simulink model "adc16x250"  (R2013b)
settings: Solver=ode45  StartTime=0.0  StopTime=10.0  RelTol=1e-3
libraries: xbsIndex_r4 x23, xps_library x1
settings Model: Creator=root  LastModifiedBy=root

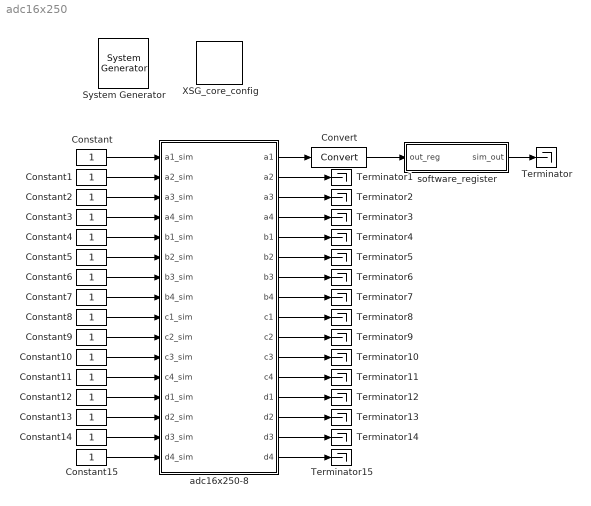
== system adc16x250 ==
  " System Generator" : xbsIndex_r4/ System Generator  Tag=genX  xilinxfamily=virtex6  part=xc6vsx475t  speed=-1  package=ff1759  synthesis_tool=XST  clock_wrapper=Clock Enables  directory=./adc16x250/sysgen  proj_type=Project Navigator  Synth_file=XST Defaults  Impl_file=ISE Defaults  testbench=off  simulink_period=1  sysclk_period=5  dcm_input_clock_period=100  incr_netlist=off  trim_vbits=Everywhere in SubSystem  dbl_ovrd=According to Block Masks  core_generation=According to Block Masks  run_coregen=off  deprecated_control=off  eval_field=0  block_type=sysgen
  Constant{,1..15} (16 alike) : Constant
  Convert : xbsIndex_r4/Convert  gui_display_data_type=Fixed-point  arith_type=Unsigned  n_bits=32  bin_pt=0  float_type=Single  exp_bits=8  fraction_bits=24  quantization=Truncate  overflow=Wrap  en=off  latency=2  dbl_ovrd=off  pipeline=off  block_type=convert
      settings: block_version=11.4
  Terminator{,1..15} (16 alike) : Terminator
  XSG_core_config : xps_library/XSG_core_config  Tag=xps:xsg  hw_sys=ROACH2:sx475t  clk_src=adc0_clk  ROACH_clk_src=sys_clk  ROACH2_clk_src=adc0_clk  MKDIG_clk_src=sys_clk  clk_rate=135  sample_period=1  synthesis_tool=XST
  adc16x250-8 : Subsystem  Tag=xps:adc16  AncestorBlock=xps_library/ADCs/adc16x250-8  mask(ADC16){board_count=1, roach2_rev=2, zdok_rev=2}
      mask prompts: board_count "Number of ADC16 Boards"; roach2_rev "ROACH2 Revision"; zdok_rev "ZDOK Pinout Revision"
      mask help: 16-input ADC. When using one ADC16 board, it must be in ZDOK0.
      mask init:
      | % Only board_count is needed by init function
      | adc16_init(gcb, ...
      |     'board_count', board_count);
      settings: AttributesFormatString=r2 rev%<roach2_rev>\nzdok rev%<zdok_rev>
      mask Help:
      | This is the CASPER "yellow block" for the CASPER ADC16 board.  Each ADC
      | board has four ADC chips.  Each ADC chip accepts four inputs.  The four
      | 8-bit outputs from each ADC chip are concatenated into a 32-bit signal.
      mask TypeOptions board_count: 1 | 2
      mask TypeOptions roach2_rev: 1 | 2
      mask TypeOptions zdok_rev: 1 | 2
  software_register : Subsystem  Tag=xps:sw_reg  AncestorBlock=xps_library/software_register  mask(swreg){io_dir=To Processor, io_delay=0, sample_period=1, names=reg, bitwidths=32, bin_pts=0, arith_types=0, sim_port=on, show_format=on}
      mask prompts: io_dir "I/O direction"; io_delay "I/O delay"; sample_period "Sample period"; names "Bitfield names [msb...lsb]"; bitwidths "Bitfield widths"; bin_pts "Bitfield binary pts"; arith_types "Bitfield types, ufix=0, fix=1, bool=2"; sim_port "Provide sim input/output?"; show_format "Print format string?"
      mask help: A 32-bit software-accessible register. Can be divided into bitfields of varying widths and types using the fields in the block mask.
      mask init:
      | try
      |     swreg_init(gcb)
      | catch ex
      |     disp(sprintf('%s: %s', gcb, ex.message))
      |     errordlg(ex.message)
      | end
      settings: AttributesFormatString=1output:uf32.0 = 32 bits
      mask TypeOptions io_dir: To Processor | From Processor
      mask Callback io_dir:
      | mask_enables = get_param(gcb, 'MaskEnables');
      | mask_names = get_param(gcb, 'MaskNames');
      | if strcmp(get_param(gcb, 'io_dir'), 'To Processor'),
      |     mask_enables{ismember(mask_names, 'sample_period')} = 'off';
      | else
      |     mask_enables{ismember(mask_names, 'sample_period')} = 'on';
      | end
      | set_param(gcb, 'MaskEnables', mask_enables);
  wires:
  adc16x250-8/1(a1) -> Convert/1
  Convert/1 -> software_register/1(out_reg)
  software_register/1(sim_out) -> Terminator/1
  adc16x250-8/2(a2) -> Terminator1/1
  adc16x250-8/3(a3) -> Terminator2/1
  adc16x250-8/4(a4) -> Terminator3/1
  adc16x250-8/5(b1) -> Terminator4/1
  adc16x250-8/6(b2) -> Terminator5/1
  adc16x250-8/7(b3) -> Terminator6/1
  adc16x250-8/8(b4) -> Terminator7/1
  adc16x250-8/9(c1) -> Terminator8/1
  adc16x250-8/10(c2) -> Terminator9/1
  adc16x250-8/11(c3) -> Terminator10/1
  adc16x250-8/12(c4) -> Terminator11/1
  adc16x250-8/13(d1) -> Terminator12/1
  adc16x250-8/14(d2) -> Terminator13/1
  adc16x250-8/15(d3) -> Terminator14/1
  adc16x250-8/16(d4) -> Terminator15/1
  Constant/1 -> adc16x250-8/1(a1_sim)
  Constant1/1 -> adc16x250-8/2(a2_sim)
  Constant3/1 -> adc16x250-8/4(a4_sim)
  Constant2/1 -> adc16x250-8/3(a3_sim)
  Constant5/1 -> adc16x250-8/6(b2_sim)
  Constant7/1 -> adc16x250-8/8(b4_sim)
  Constant6/1 -> adc16x250-8/7(b3_sim)
  Constant4/1 -> adc16x250-8/5(b1_sim)
  Constant8/1 -> adc16x250-8/9(c1_sim)
  Constant9/1 -> adc16x250-8/10(c2_sim)
  Constant11/1 -> adc16x250-8/12(c4_sim)
  Constant10/1 -> adc16x250-8/11(c3_sim)
  Constant13/1 -> adc16x250-8/14(d2_sim)
  Constant15/1 -> adc16x250-8/16(d4_sim)
  Constant14/1 -> adc16x250-8/15(d3_sim)
  Constant12/1 -> adc16x250-8/13(d1_sim)

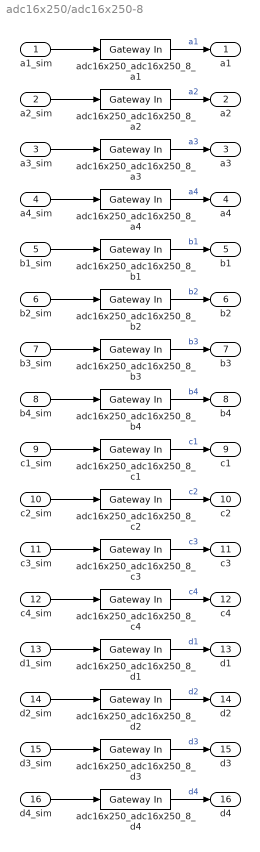
== system adc16x250/adc16x250-8 ==
  a1_sim : Inport
  a2_sim : Inport  Port=2
  a3_sim : Inport  Port=3
  a4_sim : Inport  Port=4
  b1_sim : Inport  Port=5
  b2_sim : Inport  Port=6
  b3_sim : Inport  Port=7
  b4_sim : Inport  Port=8
  c1_sim : Inport  Port=9
  c2_sim : Inport  Port=10
  c3_sim : Inport  Port=11
  c4_sim : Inport  Port=12
  d1_sim : Inport  Port=13
  d2_sim : Inport  Port=14
  d3_sim : Inport  Port=15
  d4_sim : Inport  Port=16
  adc16x250_adc16x250_8_a{1..4} (4 alike) : xbsIndex_r4/Gateway In  gui_display_data_type=Fixed-point  arith_type="Signed  (2's comp)"  n_bits=8  bin_pt=7  preci_type=Single  exp_width=8  frac_width=24  quantization="Round  (unbiased: +/- Inf)"  overflow=Saturate  period=1  dbl_ovrd=off  timing_constraint=None  locs_specified=off  LOCs={}  UseAsADC=off  ADCChannel='1'  inherit_from_input=off  hdl_port=on  block_type=gatewayin
  adc16x250_adc16x250_8_b{1..4} (4 alike) : xbsIndex_r4/Gateway In  gui_display_data_type=Fixed-point  arith_type="Signed  (2's comp)"  n_bits=8  bin_pt=7  preci_type=Single  exp_width=8  frac_width=24  quantization="Round  (unbiased: +/- Inf)"  overflow=Saturate  period=1  dbl_ovrd=off  timing_constraint=None  locs_specified=off  LOCs={}  UseAsADC=off  ADCChannel='1'  inherit_from_input=off  hdl_port=on  block_type=gatewayin
  adc16x250_adc16x250_8_c{1..4} (4 alike) : xbsIndex_r4/Gateway In  gui_display_data_type=Fixed-point  arith_type="Signed  (2's comp)"  n_bits=8  bin_pt=7  preci_type=Single  exp_width=8  frac_width=24  quantization="Round  (unbiased: +/- Inf)"  overflow=Saturate  period=1  dbl_ovrd=off  timing_constraint=None  locs_specified=off  LOCs={}  UseAsADC=off  ADCChannel='1'  inherit_from_input=off  hdl_port=on  block_type=gatewayin
  adc16x250_adc16x250_8_d{1..4} (4 alike) : xbsIndex_r4/Gateway In  gui_display_data_type=Fixed-point  arith_type="Signed  (2's comp)"  n_bits=8  bin_pt=7  preci_type=Single  exp_width=8  frac_width=24  quantization="Round  (unbiased: +/- Inf)"  overflow=Saturate  period=1  dbl_ovrd=off  timing_constraint=None  locs_specified=off  LOCs={}  UseAsADC=off  ADCChannel='1'  inherit_from_input=off  hdl_port=on  block_type=gatewayin
  a1 : Outport
  a2 : Outport  Port=2
  a3 : Outport  Port=3
  a4 : Outport  Port=4
  b1 : Outport  Port=5
  b2 : Outport  Port=6
  b3 : Outport  Port=7
  b4 : Outport  Port=8
  c1 : Outport  Port=9
  c2 : Outport  Port=10
  c3 : Outport  Port=11
  c4 : Outport  Port=12
  d1 : Outport  Port=13
  d2 : Outport  Port=14
  d3 : Outport  Port=15
  d4 : Outport  Port=16
  wires:
  a1_sim/1 -> adc16x250_adc16x250_8_a1/1
  adc16x250_adc16x250_8_a1/1 -> a1/1  "a1"
  a2_sim/1 -> adc16x250_adc16x250_8_a2/1
  adc16x250_adc16x250_8_a2/1 -> a2/1  "a2"
  a3_sim/1 -> adc16x250_adc16x250_8_a3/1
  adc16x250_adc16x250_8_a3/1 -> a3/1  "a3"
  a4_sim/1 -> adc16x250_adc16x250_8_a4/1
  adc16x250_adc16x250_8_a4/1 -> a4/1  "a4"
  b1_sim/1 -> adc16x250_adc16x250_8_b1/1
  adc16x250_adc16x250_8_b1/1 -> b1/1  "b1"
  b2_sim/1 -> adc16x250_adc16x250_8_b2/1
  adc16x250_adc16x250_8_b2/1 -> b2/1  "b2"
  b3_sim/1 -> adc16x250_adc16x250_8_b3/1
  adc16x250_adc16x250_8_b3/1 -> b3/1  "b3"
  b4_sim/1 -> adc16x250_adc16x250_8_b4/1
  adc16x250_adc16x250_8_b4/1 -> b4/1  "b4"
  c1_sim/1 -> adc16x250_adc16x250_8_c1/1
  adc16x250_adc16x250_8_c1/1 -> c1/1  "c1"
  c2_sim/1 -> adc16x250_adc16x250_8_c2/1
  adc16x250_adc16x250_8_c2/1 -> c2/1  "c2"
  c3_sim/1 -> adc16x250_adc16x250_8_c3/1
  adc16x250_adc16x250_8_c3/1 -> c3/1  "c3"
  c4_sim/1 -> adc16x250_adc16x250_8_c4/1
  adc16x250_adc16x250_8_c4/1 -> c4/1  "c4"
  d1_sim/1 -> adc16x250_adc16x250_8_d1/1
  adc16x250_adc16x250_8_d1/1 -> d1/1  "d1"
  d2_sim/1 -> adc16x250_adc16x250_8_d2/1
  adc16x250_adc16x250_8_d2/1 -> d2/1  "d2"
  d3_sim/1 -> adc16x250_adc16x250_8_d3/1
  adc16x250_adc16x250_8_d3/1 -> d3/1  "d3"
  d4_sim/1 -> adc16x250_adc16x250_8_d4/1
  adc16x250_adc16x250_8_d4/1 -> d4/1  "d4"

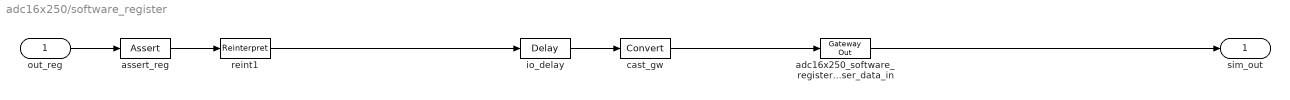
== system adc16x250/software_register ==
  out_reg : Inport
  adc16x250_software_register_user_data_in : xbsIndex_r4/Gateway Out  inherit_from_input=off  hdl_port=on  timing_constraint=None  locs_specified=off  LOCs={}  UseAsDAC=off  DACChannel='1'  block_type=gatewayout
  assert_reg : xbsIndex_r4/Assert  assert_type=on  type_source=Explicitly  gui_display_data_type=Fixed-point  arith_type=Unsigned  n_bits=32  bin_pt=0  preci_type=Single  exp_width=8  frac_width=24  assert_rate=off  rate_source=Explicitly  period=1  output_port=on  block_type=assert
  cast_gw : xbsIndex_r4/Convert  gui_display_data_type=Fixed-point  arith_type=Unsigned  n_bits=32  bin_pt=0  float_type=Single  exp_bits=8  fraction_bits=24  quantization=Truncate  overflow=Wrap  en=off  latency=0  dbl_ovrd=off  pipeline=off  block_type=convert
  io_delay : xbsIndex_r4/Delay  rst=off  infoeditControl=Selection of Reset will increase slice count due to use of real FFs and instead of SRLs  en=off  latency=0  dbl_ovrd=off  reg_retiming=on  block_type=delay
  reint1 : xbsIndex_r4/Reinterpret  force_arith_type=on  arith_type=Unsigned  force_bin_pt=on  bin_pt=0  block_type=reinterpret
  sim_out : Outport
  wires:
  io_delay/1 -> cast_gw/1
  cast_gw/1 -> adc16x250_software_register_user_data_in/1
  adc16x250_software_register_user_data_in/1 -> sim_out/1
  out_reg/1 -> assert_reg/1
  assert_reg/1 -> reint1/1
  reint1/1 -> io_delay/1
